simulink model "week3_1"  (R2020b)
settings: Solver=VariableStepAuto  StartTime=0.0  StopTime=10.0  RelTol=1e-3
settings Model: Creator=Lenovo  LastModifiedBy=Lenovo

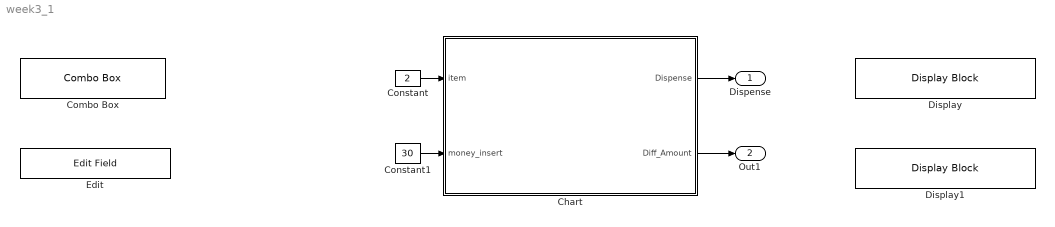
== system week3_1 ==
  Chart : Stateflow chart  TreatAsAtomicUnit=on
  Combo Box : ComboBox  LabelPosition=Hide  SelectedLabel=Water
      settings: Values={{'Coke', 'Water', 'Chocolate', 'Chips'}, [1 2 3 4]}
  Constant : Constant  Value=2
  Constant1 : Constant  Value=30
  Display : DisplayBlock  LabelPosition=Hide  Format=short  Transparency=1
  Display1 : DisplayBlock  LabelPosition=Hide  Format=short  Transparency=1
  Edit : EditField  LabelPosition=Hide  ShowInitialText=on  Alignment=Center
  Dispense : Outport  SignalName=item received
  Out1 : Outport  Port=2
  wires:
  Constant/1 -> Chart/1(item)
  Constant1/1 -> Chart/2(money_insert)
  Chart/1(Dispense) -> Dispense/1
  Chart/2(Diff_Amount) -> Out1/1

== stateflow chart week3_1/Chart ==
  state error
  state Coin_Inserted
  state Coke
  state Chips
  state Chocolate
  state water
  (junction 13) -> error [order 2] : [money_insert<18]{Dispense=0}
  (default) -> Coin_Inserted
  Coin_Inserted -> error [order 1] : [money_insert<=0]{Dispense=0}
  Coin_Inserted -> (junction 13) [order 2] : [item==1]
  (junction 13) -> Coke [order 1] : [money_insert>=18]{Dispense=1, Diff_Amount=money_insert-18}
  Coin_Inserted -> (junction 10) [order 3] : [item==2]
  Coin_Inserted -> (junction 17) [order 5] : [item==4]
  (junction 8) -> error [order 2] : [money_insert<15]{Dispense=0}
  (junction 17) -> error [order 2] : [money_insert<22]{Dispense=0}
  (junction 10) -> error [order 2] : [money_insert<20]{Dispense=0}
  Coin_Inserted -> (junction 8) [order 4] : [item==3]
  (junction 10) -> water [order 1] : [money_insert>=20]{Dispense=1, Diff_Amount=money_insert-20}
  (junction 17) -> Chips [order 1] : [money_insert>=10]{Dispense=1, Diff_Amount=money_insert-10}
  (junction 8) -> Chocolate [order 1] : [money_insert>=15]{Dispense=1, Diff_Amount=money_insert-15}
  data: item input; money_insert input; Dispense output; Diff_Amount output
